simulink model "Forward_Converter_nonideal"  (R2018a)
settings: Solver=VariableStepDiscrete  StartTime=0.0  StopTime=0.1  MaxStep=1e-4  RelTol=1e-4  EnableMultiTasking=on
libraries: powerlib x22, powerlib_meascontrol x1
Description:
  | Copyright 2008-2018 The MathWorks, Inc.
settings Model: Creator=MathWorks  LastModifiedBy=bulbu
settings SolverCC: SolverResetMethod=Robust
settings DataIOCC: ReturnWorkspaceOutputs=on
settings OptimizationCC: LifeSpan=inf
settings DebuggingCC: ReadBeforeWriteMsg=DisableAll  WriteAfterWriteMsg=DisableAll  WriteAfterReadMsg=DisableAll  MultiTaskDSMMsg=none  SFUnexpectedBacktrackingDiag=warning  SFNoUnconditionalDefaultTransitionDiag=warning  SFExecutionAtInitializationDiag=none
settings ModelReferenceCC: UpdateModelReferenceTargets=IfOutOfDate
settings SFSimCC: SFSimEcho=off
settings CodeAppCC: StateflowObjectComments=on
settings GRTTargetCC: TargetLangStandard=C89/C90 (ANSI)  GeneratePreprocessorConditionals=Disable all
settings ConfigComp: CovMetricSettings=dw  CovHtmlReporting=on  CovSaveCumulativeToWorkspaceVar=on  CovSaveSingleToWorkspaceVar=on  CovExternalEMLEnable=off
settings SimscapeCC: SimscapeNormalizeSystem=off  SimscapeNominalValues={1, 'bar'; 1, 'cm^3/s'; 1, 'bar*kg/s'; 1, 'kJ/kg'; 1, 'kW'; }

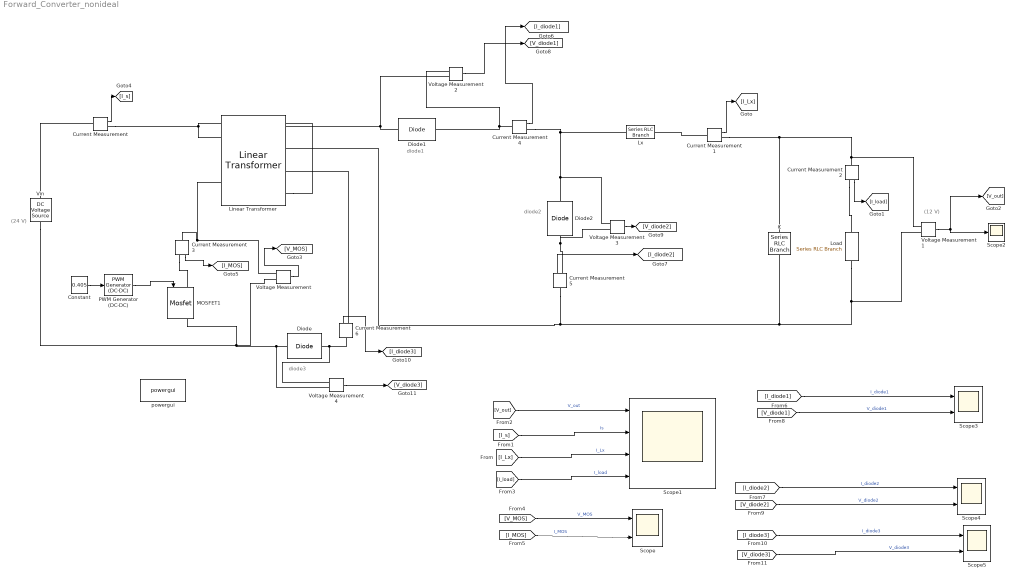
== system Forward_Converter_nonideal ==
  note: diode1
  note: (12 V)
  note: (24 V)
  note: diode2
  note: diode3
  C : powerlib/Elements/Series RLC Branch  LConnTagsString=__new0  RConnTagsString=__new0  BranchType=C  Resistance=1e-4  Inductance=200e-6  SetiL0=off  InitialCurrent=0  Capacitance=100e-6  Setx0=off  InitialVoltage=0  Measurements=None
  Constant : Constant  Value=0.405
  Current Measurement{,1..6} (7 alike) : powerlib/Measurements/Current Measurement  PhasorSimulation=off  OutputType=Complex  PSBequivalent=0
  Diode : powerlib/Power Electronics/Diode  Ron=0.001  Lon=0  Vf=0.78  IC=0  UseSnubber=0  Rs=500  Cs=250e-9  Measurements=off
  Diode1 : powerlib/Power Electronics/Diode  Ron=17.7e-3  Lon=0  Vf=0.78  IC=0  UseSnubber=0  Rs=500  Cs=250e-9  Measurements=off
  Diode2 : powerlib/Power Electronics/Diode  Ron=0.001  Lon=0  Vf=0.78  IC=0  UseSnubber=0  Rs=500  Cs=250e-9  Measurements=off
  Linear Transformer : powerlib/Elements/Linear Transformer  UNITS=SI  NominalPower=[ 25 31.25e3 ]  winding1=[15 0.0219 0.9e-06]  winding2=[20 0.0331 0.9e-06]  ThreeWindings=on  winding3=[15 5e-03 1e-06]  RmLm=[500 0.66e-3]  Measurements=Magnetization current  DataType=on
  Load : powerlib/Elements/Series RLC Branch  LConnTagsString=__new0  RConnTagsString=__new0  BranchType=R  Resistance=2.87  Inductance=200e-6  SetiL0=off  InitialCurrent=0  Capacitance=400e-6  Setx0=off  InitialVoltage=0  Measurements=Branch current
  Lx : powerlib/Elements/Series RLC Branch  LConnTagsString=__new0  RConnTagsString=__new0  BranchType=L  Resistance=10  Inductance=200e-6  SetiL0=off  InitialCurrent=0  Capacitance=400e-6  Setx0=off  InitialVoltage=0  Measurements=Branch current
  MOSFET1 : powerlib/Power Electronics/Mosfet  Ron=0.27  Lon=0  Rd=1e-3  Vfd=1.4  IC=0  Rs=1e6  Cs=inf  Measurements=on
  PWM Generator (DC-DC) : powerlib_meascontrol/Pulse & Signal Generators/PWM Generator (DC-DC)  Fsw=35000  Ts=0
  Scope{,3..5} (4 alike) : Scope  NumInputPorts=2
  Scope1 : Scope  NumInputPorts=4
  Scope2 : Scope
  Vin : powerlib/Electrical Sources/DC Voltage Source  Amplitude=24  Measurements=None
  Voltage Measurement{,1..4} (5 alike) : powerlib/Measurements/Voltage Measurement  PhasorSimulation=off  OutputType=Complex  PSBequivalent=0
  powergui : powerlib/powergui  Priority=1  SimulationMode=Discrete  SampleTime=1e-6  frequency=60  Iterations=50  frequencyindice=0  Pbase=100e6  ErrMax=1e-4  UnitsV=kV  UnitsW=MW  buscounter=0  FunctionMessages=off  echomessages=off  EnableUseOfTLC=off  CurrentSourceSwitches=off  DisableSnubberDevices=off  DisableRonSwitches=off  DisableVfSwitches=off  DisplayEquations=off  SolverType=Tustin/Backward Euler (TBE)  Interpol=off  ExternalGateDelay=off  methode=off  Ts=100  x0status=blocks  SPID=on  SwTol=0  HookPort=off  RestoreLinks=warning  ResistiveCurrentMeasurement=off  Frange=[0:2:500]  Ylog=off  Xlog=on  ShowGrid=off  save=off  variable=ZData  structure=0  ZoomFFT=off  StartTime=0.0  cycles=1  DisplayStyle=1  fundamental=60  FreqAxis=off  MaxFrequency=1000  frequencyindicesteady=1  RmsSteady=1  display=off
  wires:
  Voltage Measurement1/1 -> [V_out], Scope2/1
  Current Measurement/1 -> [I_s]
  [I_s] -> Scope1/2  "Is"
  Current Measurement1/1 -> [I_Lx]
  Current Measurement2/1 -> [I_load]
  [I_Lx] -> Scope1/3  "I_Lx"
  [I_load] -> Scope1/4  "I_load"
  [V_out] -> Scope1/1  "V_out"
  Constant/1 -> PWM Generator (DC-DC)/1
  Voltage Measurement/1 -> [V_MOS]
  [V_MOS] -> Scope/1  "V_MOS"
  Current Measurement3/1 -> [I_MOS]
  [I_MOS] -> Scope/2  "I_MOS"
  Current Measurement4/1 -> [I_diode1]
  [I_diode1] -> Scope3/1  "I_diode1"
  [V_diode1] -> Scope3/2  "V_diode1"
  [I_diode2] -> Scope4/1  "I_diode2"
  [V_diode2] -> Scope4/2  "V_diode2"
  Current Measurement5/1 -> [I_diode2]
  Voltage Measurement2/1 -> [V_diode1]
  Voltage Measurement3/1 -> [V_diode2]
  PWM Generator (DC-DC)/1 -> MOSFET1/1
  Current Measurement6/1 -> [I_diode3]
  Voltage Measurement4/1 -> [V_diode3]
  [I_diode3] -> Scope5/1  "I_diode3"
  [V_diode3] -> Scope5/2  "V_diode3"
  connections:
  Current Measurement1/RConn1 -- Voltage Measurement1/LConn1 -- Current Measurement2/LConn1 -- C/LConn1
  Load/RConn1 -- Voltage Measurement1/LConn2 -- Linear Transformer/RConn2 -- Current Measurement5/LConn1 -- C/RConn1
  Voltage Measurement/LConn1 -- Current Measurement3/LConn1 -- Linear Transformer/LConn2
  Vin/LConn1 -- MOSFET1/RConn1 -- Voltage Measurement4/LConn2 -- Diode/LConn1 -- Voltage Measurement/LConn2
  Linear Transformer/RConn4 -- Current Measurement/RConn1 -- Linear Transformer/LConn1
  Diode1/LConn1 -- Voltage Measurement2/LConn2 -- Linear Transformer/RConn1
  Diode2/RConn1 -- Voltage Measurement3/LConn1 -- Current Measurement4/RConn1 -- Lx/LConn1
  Vin/RConn1 -- Current Measurement/LConn1
  Current Measurement1/LConn1 -- Lx/RConn1
  Current Measurement2/RConn1 -- Load/LConn1
  Current Measurement3/RConn1 -- MOSFET1/LConn1
  Current Measurement4/LConn1 -- Voltage Measurement2/LConn1 -- Diode1/RConn1
  Current Measurement5/RConn1 -- Voltage Measurement3/LConn2 -- Diode2/LConn1
  Diode/RConn1 -- Voltage Measurement4/LConn1 -- Current Measurement6/LConn1
  Current Measurement6/RConn1 -- Linear Transformer/RConn3
